simulink model "traffic_light_controller"  (R2015b)
settings: Solver=VariableStepAuto  StartTime=0.0  StopTime=inf  RelTol=1e-3
libraries: arduinolib x13
settings Model: Creator=Monty  LastModifiedBy=Monty

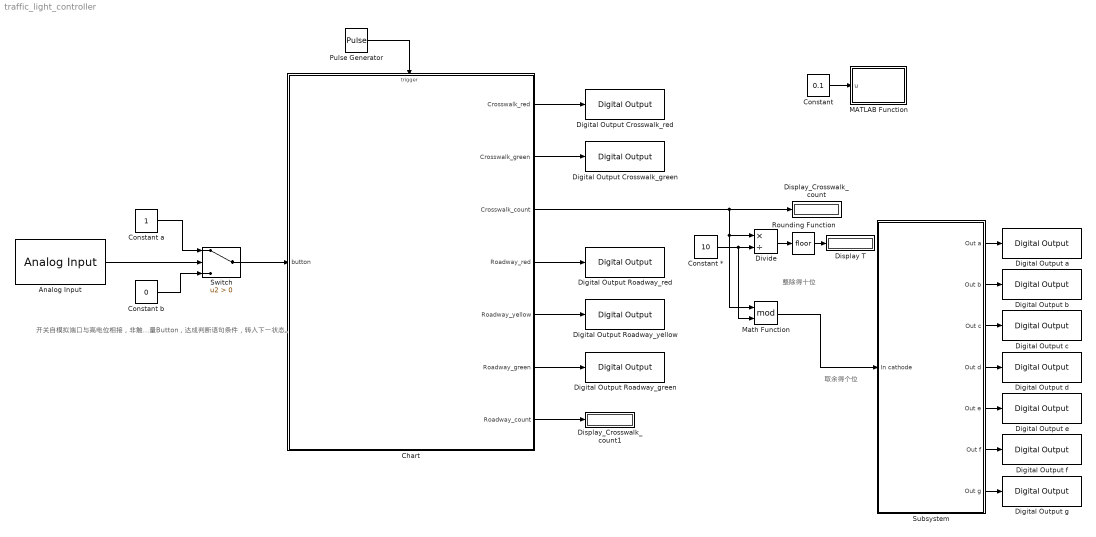
== system traffic_light_controller ==
  note: 开关自模拟端口与高电位相接，非触发状态下呈低电位，经Switch判断后将常数1赋值给变量Button；开关触发后呈高电位，经Switch判断后将常数0赋值给变量Button，达成判断语句条件，转入下一状态。
  note: 整除得十位
  note: 取余得个位
  Analog Input : arduinolib/Analog Input  pinNumber=1  sampleTime=0.5  blockPlatform=arduino
  Chart : Stateflow chart  TreatAsAtomicUnit=on
  Constant : Constant  Value=0.1
  Constant * : Constant  Value=10
  Constant a : Constant
  Constant b : Constant  Value=0
  Digital Output Crosswalk_green : arduinolib/Digital Output  pinNumber=10  blockPlatform=arduino
  Digital Output Crosswalk_red : arduinolib/Digital Output  pinNumber=9  blockPlatform=arduino
  Digital Output Roadway_green : arduinolib/Digital Output  pinNumber=13  blockPlatform=arduino
  Digital Output Roadway_red : arduinolib/Digital Output  pinNumber=11  blockPlatform=arduino
  Digital Output Roadway_yellow : arduinolib/Digital Output  pinNumber=12  blockPlatform=arduino
  Digital Output a : arduinolib/Digital Output  pinNumber=2  blockPlatform=arduino
  Digital Output b : arduinolib/Digital Output  pinNumber=3  blockPlatform=arduino
  Digital Output c : arduinolib/Digital Output  pinNumber=4  blockPlatform=arduino
  Digital Output d : arduinolib/Digital Output  pinNumber=5  blockPlatform=arduino
  Digital Output e : arduinolib/Digital Output  pinNumber=6  blockPlatform=arduino
  Digital Output f : arduinolib/Digital Output  pinNumber=7  blockPlatform=arduino
  Digital Output g : arduinolib/Digital Output  pinNumber=8  blockPlatform=arduino
  Display T : Display
  Display_Crosswalk_count : Display
  Display_Crosswalk_count1 : Display
  Divide : Product  Inputs=*/
  MATLAB Function : MATLAB Function  TreatAsAtomicUnit=on
  Math Function : Math  Operator=mod  SaturateOnIntegerOverflow=on
  Pulse Generator : DiscretePulseGenerator  PulseType=Time based  Period=1  PulseWidth=50
  Rounding Function : Rounding
  Subsystem : Subsystem
      mask Display:
      | disp('七段数码管驱动模块\n信息1901邱剑楠')
      | port_label('input',1,'输入')
      | port_label('output',1,'a(2)')
      | port_label('output',2,'b(3)')
      | port_label('output',3,'c(4)')
      | port_label('output',4,'d(5)')
      | port_label('output',5,'e(6)')
      | port_label('output',6,'f(7)')
      | port_label('output',7,'g(8)')
  Switch : Switch  Criteria=u2 > Threshold
  wires:
  Chart/1(Crosswalk_red) -> Digital Output Crosswalk_red/1
  Chart/2(Crosswalk_green) -> Digital Output Crosswalk_green/1
  Chart/4(Roadway_red) -> Digital Output Roadway_red/1
  Chart/5(Roadway_yellow) -> Digital Output Roadway_yellow/1
  Chart/6(Roadway_green) -> Digital Output Roadway_green/1
  Chart/3(Crosswalk_count) -> Divide/1, Math Function/1, Display_Crosswalk_count/1
  Constant */1 -> Math Function/2, Divide/2
  Divide/1 -> Rounding Function/1
  Math Function/1 -> Subsystem/1(In cathode)
  Subsystem/1(Out a) -> Digital Output a/1
  Subsystem/2(Out b) -> Digital Output b/1
  Subsystem/3(Out c) -> Digital Output c/1
  Subsystem/4(Out d) -> Digital Output d/1
  Subsystem/5(Out e) -> Digital Output e/1
  Subsystem/6(Out f) -> Digital Output f/1
  Subsystem/7(Out g) -> Digital Output g/1
  Rounding Function/1 -> Display T/1
  Chart/7(Roadway_count) -> Display_Crosswalk_count1/1
  Pulse Generator/1 -> Chart/Trigger
  Constant/1 -> MATLAB Function/1(u)
  Analog Input/1 -> Switch/2
  Switch/1 -> Chart/1(button)
  Constant a/1 -> Switch/1
  Constant b/1 -> Switch/3

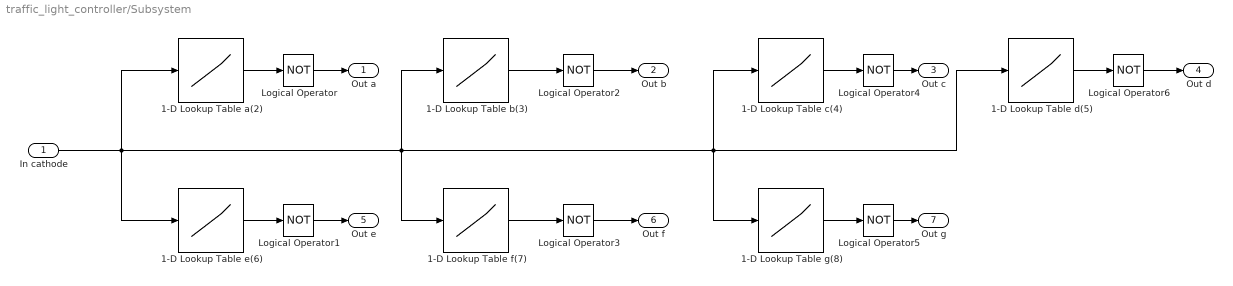
== system traffic_light_controller/Subsystem ==
  In cathode : Inport
  1-D Lookup Table a(2) : Lookup_n-D  NumberOfTableDimensions=1  BreakpointsForDimension1=[0 1 2 3 4 5 6 7 8 9]  BreakpointsForDimension1FirstPoint=10  BreakpointsForDimension2FirstPoint=10  BreakpointsForDimension1Spacing=12  BreakpointsForDimension2Spacing=12  IndexSearchMethod=Evenly spaced points  Table=[1 0 1 1 0 1 1 1 1 1]  InterpMethod=Flat  DiagnosticForOutOfRangeInput=Error  InternalRulePriority=Speed  RndMeth=Simplest  InputSameDT=on
  1-D Lookup Table b(3) : Lookup_n-D  NumberOfTableDimensions=1  BreakpointsForDimension1=[0 1 2 3 4 5 6 7 8 9]  BreakpointsForDimension1FirstPoint=10  BreakpointsForDimension2FirstPoint=10  BreakpointsForDimension1Spacing=12  BreakpointsForDimension2Spacing=12  IndexSearchMethod=Evenly spaced points  Table=[1 1 1 1 1 0 0 1 1 1]  InterpMethod=Flat  DiagnosticForOutOfRangeInput=Error  InternalRulePriority=Speed  RndMeth=Simplest  InputSameDT=on
  1-D Lookup Table c(4) : Lookup_n-D  NumberOfTableDimensions=1  BreakpointsForDimension1=[0 1 2 3 4 5 6 7 8 9]  BreakpointsForDimension1FirstPoint=10  BreakpointsForDimension2FirstPoint=10  BreakpointsForDimension1Spacing=12  BreakpointsForDimension2Spacing=12  IndexSearchMethod=Evenly spaced points  Table=[1 1 0 1 1 1 1 1 1 1]  InterpMethod=Flat  DiagnosticForOutOfRangeInput=Error  InternalRulePriority=Speed  RndMeth=Simplest  InputSameDT=on
  1-D Lookup Table d(5) : Lookup_n-D  NumberOfTableDimensions=1  BreakpointsForDimension1=[0 1 2 3 4 5 6 7 8 9]  BreakpointsForDimension1FirstPoint=10  BreakpointsForDimension2FirstPoint=10  BreakpointsForDimension1Spacing=12  BreakpointsForDimension2Spacing=12  IndexSearchMethod=Evenly spaced points  Table=[1 0 1 1 0 1 1 0 1 1]  InterpMethod=Flat  DiagnosticForOutOfRangeInput=Error  InternalRulePriority=Speed  RndMeth=Simplest  InputSameDT=on
  1-D Lookup Table e(6) : Lookup_n-D  NumberOfTableDimensions=1  BreakpointsForDimension1=[0 1 2 3 4 5 6 7 8 9]  BreakpointsForDimension1FirstPoint=10  BreakpointsForDimension2FirstPoint=10  BreakpointsForDimension1Spacing=12  BreakpointsForDimension2Spacing=12  IndexSearchMethod=Evenly spaced points  Table=[1 0 1 0 0 0 1 0 1 0]  InterpMethod=Flat  DiagnosticForOutOfRangeInput=Error  InternalRulePriority=Speed  RndMeth=Simplest  InputSameDT=on
  1-D Lookup Table f(7) : Lookup_n-D  NumberOfTableDimensions=1  BreakpointsForDimension1=[0 1 2 3 4 5 6 7 8 9]  BreakpointsForDimension1FirstPoint=10  BreakpointsForDimension2FirstPoint=10  BreakpointsForDimension1Spacing=12  BreakpointsForDimension2Spacing=12  IndexSearchMethod=Evenly spaced points  Table=[1 0 0 0 1 1 1 0 1 1]  InterpMethod=Flat  DiagnosticForOutOfRangeInput=Error  InternalRulePriority=Speed  RndMeth=Simplest  InputSameDT=on
  1-D Lookup Table g(8) : Lookup_n-D  NumberOfTableDimensions=1  BreakpointsForDimension1=[0 1 2 3 4 5 6 7 8 9]  BreakpointsForDimension1FirstPoint=10  BreakpointsForDimension2FirstPoint=10  BreakpointsForDimension1Spacing=12  BreakpointsForDimension2Spacing=12  IndexSearchMethod=Evenly spaced points  Table=[0 0 1 1 1 1 1 0 1 1]  InterpMethod=Flat  DiagnosticForOutOfRangeInput=Error  InternalRulePriority=Speed  RndMeth=Simplest  InputSameDT=on
  Logical Operator{,1..6} (7 alike) : Logic  Operator=NOT  AllPortsSameDT=off  OutDataTypeStr=boolean
  Out a : Outport
  Out b : Outport  Port=2
  Out c : Outport  Port=3
  Out d : Outport  Port=4
  Out e : Outport  Port=5
  Out f : Outport  Port=6
  Out g : Outport  Port=7
  wires:
  1-D Lookup Table a(2)/1 -> Logical Operator/1
  1-D Lookup Table g(8)/1 -> Logical Operator5/1
  1-D Lookup Table f(7)/1 -> Logical Operator3/1
  In cathode/1 -> 1-D Lookup Table e(6)/1, 1-D Lookup Table a(2)/1, 1-D Lookup Table f(7)/1, 1-D Lookup Table b(3)/1, 1-D Lookup Table g(8)/1, 1-D Lookup Table d(5)/1, 1-D Lookup Table c(4)/1
  1-D Lookup Table b(3)/1 -> Logical Operator2/1
  1-D Lookup Table e(6)/1 -> Logical Operator1/1
  1-D Lookup Table d(5)/1 -> Logical Operator6/1
  1-D Lookup Table c(4)/1 -> Logical Operator4/1
  Logical Operator/1 -> Out a/1
  Logical Operator1/1 -> Out e/1
  Logical Operator2/1 -> Out b/1
  Logical Operator3/1 -> Out f/1
  Logical Operator4/1 -> Out c/1
  Logical Operator5/1 -> Out g/1
  Logical Operator6/1 -> Out d/1

== matlab function traffic_light_controller/MATLAB Function ==
  data: u input
function fcn(u)
%#codegen

pause(u);

== stateflow chart traffic_light_controller/Chart ==
  state State2
    entry:Crosswalk_red=1;
    Crosswalk_green=0;
    Roadway_red=0;
    Roadway_green=0;
    Led_num=6;
    Crosswalk_count=Led_num;
    Roadway_count=Led_num;
    state State2_2
      entry:Roadway_yellow=0;
    state State2_1
      entry:Roadway_yellow=1;
    (default) -> State2_1
    State2_1 -> State2_2 : after(1,sec)
    State2_2 -> State2_1 : after(1,sec)
  state State1
    entry:Crosswalk_red=1;
    Crosswalk_green=0;
    Roadway_red=0;
    Roadway_yellow=0;
    Roadway_green=1;
  note: 倒计时模块，每经过一个内部时间脉冲TIC，倒计时所用参数减一
  state State4
    entry:Crosswalk_red=0;
    Roadway_red=1;
    Roadway_yellow=0;
    Roadway_green=0;
    Led_num=10;
    Crosswalk_count=Led_num;
    Roadway_count=Led_num;
    state State4_2
      entry:Crosswalk_green=0;
    state State4_1
      entry:Crosswalk_green=1;
    (default) -> State4_1
    State4_1 -> State4_2 : after(1,sec)
    State4_2 -> State4_1 : after(1,sec)
  state State3
    entry:Crosswalk_red=0;
    Crosswalk_green=1;
    Roadway_red=1;
    Roadway_yellow=0;
    Roadway_green=0;
    Led_num=10;
    Crosswalk_count=Led_num+10;
    Roadway_count=Led_num+10;
  (default) -> State1
  State1 -> State2 : [button==0]
  State4 -> State1 [order 1] : after(Led_num,sec)
  State2 -> (junction 27) [order 2] : TIC
  State2 -> State3 [order 1] : after(Led_num,sec)
  (junction 27) -> (junction 32) : {Crosswalk_count=Crosswalk_count-1;
      | Roadway_count=Roadway_count-1;}
  State4 -> (junction 27) [order 2] : TIC
  State3 -> (junction 27) [order 2] : TIC
  State3 -> State4 [order 1] : after(Led_num,sec)
  data: Crosswalk_red output; Crosswalk_green output; Crosswalk_count output; Roadway_red output; Roadway_yellow output; Roadway_green output; Led_num local; Roadway_count output; button input
  events: TIC input RISING_EDGE_EVENT
